simulink model "vccmspex"  (Simulink 3.00)
settings: Solver=FixedStepDiscrete  StartTime=0.0  StopTime=10.0  RelTol=1e-3
libraries: simulink3 x4, smxl x4
settings Model: LastModifiedBy=giampiero

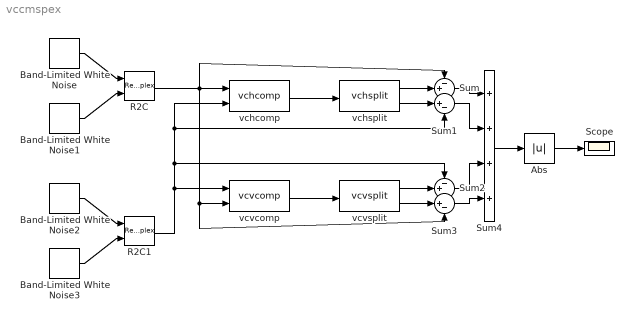
== system vccmspex ==
  Abs : Abs
  Band-Limited White Noise : simulink3/Sources/Band-Limited White Noise  Cov=[0.1]*ones(6,1)  Ts=0.1  seed=1:6
  Band-Limited White Noise1 : simulink3/Sources/Band-Limited White Noise  Cov=[0.1]*ones(6,1)  Ts=0.1  seed=7:12
  Band-Limited White Noise2 : simulink3/Sources/Band-Limited White Noise  Cov=[0.1]*ones(6,1)  Ts=0.1  seed=12+[1:6]
  Band-Limited White Noise3 : simulink3/Sources/Band-Limited White Noise  Cov=[0.1]*ones(6,1)  Ts=0.1  seed=18+[1:6]
  R2C : RealImagToComplex  Input=RealAndImag  ConstantPart=0
  R2C1 : RealImagToComplex  Input=RealAndImag  ConstantPart=0
  Scope : Scope
      settings: TickLabels=on  TimeRange=10  YMin=-1e-016  YMax=1e-016  SaveToWorkspace=off  SaveName=ScopeData
  Sum : Sum  Inputs=-+|  SaturateOnIntegerOverflow=on
  Sum1 : Sum  Inputs=|+-  SaturateOnIntegerOverflow=on
  Sum2 : Sum  Inputs=-+|  SaturateOnIntegerOverflow=on
  Sum3 : Sum  Inputs=|+-  SaturateOnIntegerOverflow=on
  Sum4 : Sum  Inputs=4  SaturateOnIntegerOverflow=on
  vchcomp : smxl/Complex Matrices/vchcomp  dims=[3 2 2]
  vchsplit : smxl/Complex Matrices/vchsplit  dims=[3 2 2]
  vcvcomp : smxl/Complex Matrices/vcvcomp  dims=[3 3 2]
  vcvsplit : smxl/Complex Matrices/vcvsplit  dims=[3 3 2]
  wires:
  Band-Limited White Noise/1 -> R2C/1
  Band-Limited White Noise1/1 -> R2C/2
  Band-Limited White Noise2/1 -> R2C1/1
  Band-Limited White Noise3/1 -> R2C1/2
  R2C/1 -> vchcomp/1, Sum/1, vcvcomp/2, Sum3/2
  vchcomp/1 -> vchsplit/1
  vcvcomp/1 -> vcvsplit/1
  vchsplit/1 -> Sum/2
  vchsplit/2 -> Sum1/1
  vcvsplit/1 -> Sum2/2
  vcvsplit/2 -> Sum3/1
  R2C1/1 -> vcvcomp/1, vchcomp/2, Sum1/2, Sum2/1
  Sum/1 -> Sum4/1
  Sum1/1 -> Sum4/2
  Sum2/1 -> Sum4/3
  Sum3/1 -> Sum4/4
  Sum4/1 -> Abs/1
  Abs/1 -> Scope/1
